simulink library "visionutilities"  (R2015b)
settings: Solver=ode45  SolverMode=SingleTasking  StartTime=0.0  StopTime=10.0  RelTol=1e-3
values from neighbouring files (symbols this model uses):
  M = [row_scores', col_scores]    [cvalgMatchFeatures.m]    (also in extrinsics.m = size(imagePoints, 1); invertedImageIndex.m = size(features, 1))
  N = int32(ceil(num/den))    [estimateGeometricTransform.m]
  sz = int32(imageSize)    [detectMSERFeatures.m]    (also in detectSURFFeatures.m = size(Iu8); extractFeatures.m = [NaN 2]; imageCategoryClassifier.m = numel(colHeading))
libraries: vipmisc x3
settings Model: FPTRunName=Active  ExtModeAutoUpdateStatusClock=off  Creator=The MathWorks, Inc.  LastModifiedBy=The MathWorks, Inc.
settings DataIOCC: SaveFormat=Array  SignalLoggingSaveFormat=ModelDataLogs
settings OptimizationCC: BlockReduction=off  BooleanDataType=off  ExpressionDepthLimit=2147483647
settings DebuggingCC: SaveWithParameterizedLinksMsg=none  UnderspecifiedInitializationDetection=Classic  MergeDetectMultiDrivingBlocksExec=none  SignalResolutionControl=TryResolveAllWithWarning  FcnCallInpInsideContextMsg=UseLocalSettings  StateNameClashWarn=warning  StrictBusMsg=Warning
settings HardwareCC: ProdBitPerPointer=32  ProdLargestAtomicFloat=None  ProdIntDivRoundTo=Undefined  ProdEndianess=Unspecified  ProdWordSize=32  ProdHWDeviceType=32-bit Generic  TargetUnknown=on
settings GRTTargetCC: GeneratePreprocessorConditionals=Disable all  CombineOutputUpdateFcns=off  GRTInterface=on
settings ConfigComp: CovModelRefEnable=Off

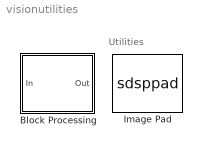
== system visionutilities ==
  note: Utilities
  Block Processing : Subsystem  DialogController=vipDDGCreate  TreatAsAtomicUnit=on  mask(Block Processing){NumI=1, ParamPort=off, NumO=1, Blocksize={[8 8]}, Overlapsize={[0 0]}, Traverse=Row-wise}
      mask prompts: NumI "Number of inputs:"; ParamPort "Add port to supply subsystem parameters"; NumO "Number of outputs:"; Blocksize "Block size:"; Overlapsize "Overlap size:"; Traverse "Order of traversing:"
      mask help:
      | Repeats a user-specified operation on submatrices of the input matrix.
      |
      | This block extracts submatrices of a user-specified size from the input matrix. It sends each submatrix to a subsystem for processing, and then reassembles each subsystem output into the output matrix.
      |
      | Use the Block size and Overlap parameters to specify the size and overlap of each submatrix in cell array format.
      mask init:
      | errmsg = vipblkblockproc(gcbh, NumI, NumO, Blocksize, Overlapsize, Traverse, ParamPort);
      | error(errmsg);
      settings: CopyFcn=set_param(gcb,'LinkStatus','none');
      mask Help: eval('helpview(fullfile(docroot,''toolbox'',''vision'',''vision.map''),''visionblockprocessing'')');
      mask TypeOptions Traverse: Row-wise | Column-wise
      mask Display:
      | disp('Block\n Processing');
      | 
      | if ((NumI == 1) && ParamPort)
      |     port_label('input', 1, 'I');
      | end
      | 
      | if (NumI > 1)
      |     for (i = 1:NumI)
      |         port_label('input', i, ['I' int2str(i)]);
      |     end
      | end
      | 
      | if (ParamPort)
      |     port_label('input', NumI+1, 'P');
      | end
  Image Pad : S-Function  FunctionName=sdsppad  Parameters=method,valSrc,value,spec,outColsMode,rowDirection,rowSize,outColSize,outRowsMode,colDirection,colSize,outRowSize,trunc_flag,0,0,0,0,0,0,0,2  SFunctionDeploymentMode=off  EnableBusSupport=on  mask(Image Pad){method=Constant, valSrc=Specify via dialog, value=0, spec=Pad size, rowDirection=Both left and right, outRowsMode=User-specified, rowSize=2, outColSize=10, colDirection=Both top and bottom, outColsMode=User-specified, colSize=[2 3], outRowSize=12, trunc_flag=None}
      mask prompts: valSrc "Pad value source:"; value "Pad value:"; spec "Specify:"; rowDirection "Add columns to:"; outRowsMode "Output row mode:"; rowSize "Number of added columns:"; outColSize "Number of output columns:"; colDirection "Add rows to:"; outColsMode "Output column mode:"; colSize "Number of added rows:"; outRowSize "Number of output rows:"; trunc_flag "Action when truncation occurs:"
      mask help:
      | Pad a two-dimensional image.
      |
      | Pad your image by adding rows, columns, or rows and columns.  You can pad your image by using a constant value, repeating its border values, using its mirror image, or using circular repetition of its elements.
      mask init:
      | ports = vipblk2dpad('icon');
      mask Help: eval('visionblockhelp');
      mask TypeOptions method: Constant | Replicate | Symmetric | Circular
      mask Callback method: vipblk2dpad
      mask TypeOptions valSrc: Specify via dialog | Input port
      mask Callback valSrc: vipblk2dpad
      mask TypeOptions spec: Pad size | Output size
      mask Callback spec: vipblk2dpad
      mask TypeOptions rowDirection: Left | Right | Both left and right | No padding
      mask Callback rowDirection: vipblk2dpad
      mask TypeOptions outRowsMode: User-specified | Next power of two
      mask Callback outRowsMode: vipblk2dpad
      mask TypeOptions colDirection: Top | Bottom | Both top and bottom | No padding
      mask Callback colDirection: vipblk2dpad
      mask TypeOptions outColsMode: User-specified | Next power of two
      mask Callback outColsMode: vipblk2dpad
      mask TypeOptions trunc_flag: None | Warning | Error
      mask Display:
      | disp('Image Pad');
      | port_label('input',ports.port1, ports.txt1);
      | port_label('input',ports.port2, ports.txt2);
      | port_label('output',ports.port3, ports.txt3);

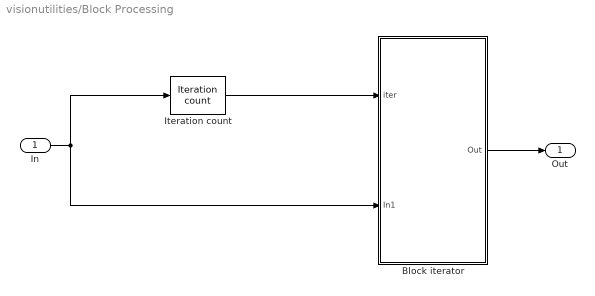
== system visionutilities/Block Processing ==
  In : Inport
  Block iterator : Subsystem
      settings: CopyFcn=set_param(gcb,'ReferenceBlock','');
  Iteration count : vipmisc/Iteration count  NumI=NumI  blksize=Blocksize  ovlpsize=Overlapsize
  Out : Outport
  wires:
  Block iterator/1(Out) -> Out/1
  In/1 -> Block iterator/2(In1), Iteration count/1
  Iteration count/1 -> Block iterator/1(iter)

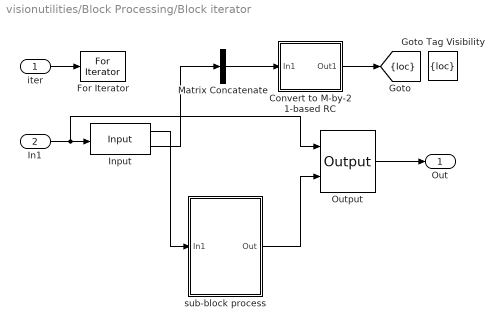
== system visionutilities/Block Processing/Block iterator ==
  iter : Inport
  In1 : Inport  Port=2
  Convert to M-by-2 1-based RC : Subsystem
  For Iterator : ForIterator  IterationSource=external  IterationLimit=(sz(1)/M)*(sz(2)/N)  ShowIterationPort=off  IndexMode=Zero-based  IterationVariableDataType=double
  Goto Tag Visibility : GotoTagVisibility  GotoTag=loc
  Input : vipmisc/Input  Blocksize=Blocksize{1}  Overlapsize=Overlapsize{1}  tverse=Row-wise
  Matrix Concatenate : Concatenate  NumInputs=1  Mode=Multidimensional array  ConcatenateDimension=2
  Output : vipmisc/Output  Blocksize=Blocksize{1}  Overlapsize=Overlapsize{1}  tverse=Row-wise
  sub-block process : Subsystem
  Out : Outport
  tag scope: loc=scoped
  wires:
  sub-block process/1(Out) -> Output/2
  Output/1 -> Out/1
  In1/1 -> Output/1, Input/1
  iter/1 -> For Iterator/1
  Input/1 -> sub-block process/1(In1)
  Input/2 -> Matrix Concatenate/1
  Matrix Concatenate/1 -> Convert to M-by-2 1-based RC/1(In1)
  Convert to M-by-2 1-based RC/1(Out1) -> [loc]

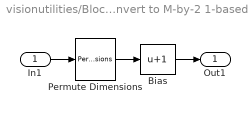
== system visionutilities/Block Processing/Block iterator/Convert to M-by-2 1-based RC ==
  In1 : Inport
  Bias : Bias  Bias=1
  Permute Dimensions : PermuteDimensions
  Out1 : Outport
  wires:
  Permute Dimensions/1 -> Bias/1
  Bias/1 -> Out1/1
  In1/1 -> Permute Dimensions/1

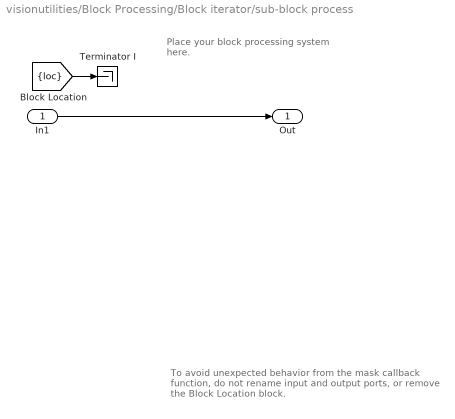
== system visionutilities/Block Processing/Block iterator/sub-block process ==
  note: Place your block
      | processing system here.
  note: To avoid unexpected behavior from the mask
      | callback function, do not rename input and output ports,
      | or remove the Block Location block.
  In1 : Inport
  Terminator I : Terminator
  Out : Outport
  wires:
  In1/1 -> Out/1
  [loc] -> Terminator I/1
